simulink model "accum_rst2"  (Simulink 6.3)
settings: Solver=ode45  StartTime=0.0  StopTime=10.0  RelTol=1e-3
settings Model: LastModifiedBy=jwallace

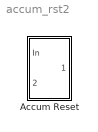
== system accum_rst2 ==
  Accum Reset : Subsystem

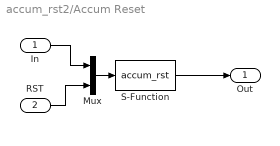
== system accum_rst2/Accum Reset ==
  In : Inport
  RST : Inport  Port=2
  Mux : Mux  Inputs=2
  S-Function : S-Function  FunctionName=accum_rst
  Out : Outport
  wires:
  S-Function/1 -> Out/1
  Mux/1 -> S-Function/1
  In/1 -> Mux/1
  RST/1 -> Mux/2
